simulink model "zbiornik1"  (R2015a)
settings: Solver=ode3  StartTime=0.0  StopTime=50  FixedStep=0.01  RelTol=1e-3
values from neighbouring files (symbols this model uses):
  a = 35    [ident1.m]    (also in wyniki_akt.mat; zbiornik_1.m; zbiornik_2.m; zbiornik_3.m)
  a1 = x(2)    [ident1.m]    (also in wyniki_akt.mat = 0.5)
  C1 = x(1)    [ident1.m]    (also in wyniki_akt.mat = 30)
  h10 = max(y1)    [ucinanie.m]
  w = 5    [ident1.m]    (also in wyniki_akt.mat; zbiornik_1.m; zbiornik_2.m; zbiornik_3.m)
settings Model: Creator=Ziger  LastModifiedBy=Student

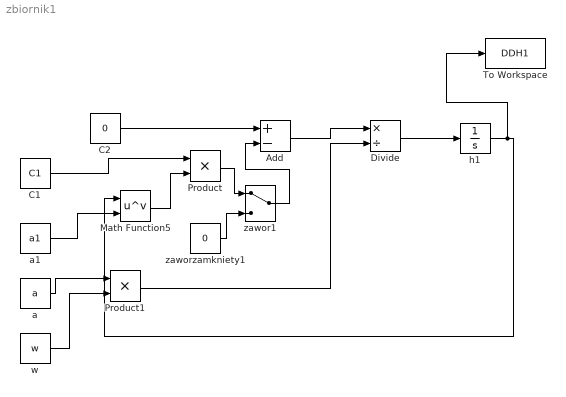
== system zbiornik1 ==
  Add : Sum  Inputs=+-
  C1 : Constant  Value=C1
  C2 : Constant  Value=0
  Divide : Product  Inputs=*/
  Math Function5 : Math  Operator=pow  SaturateOnIntegerOverflow=on
  Product : Product
  Product1 : Product
  To Workspace : ToWorkspace  VariableName=DDH1  SaveFormat=Structure With Time  SampleTime=-1
  a : Constant  Value=a
  a1 : Constant  Value=a1
  h1 : Integrator  InitialCondition=h10  LimitOutput=on  UpperSaturationLimit=35  LowerSaturationLimit=0
  w : Constant  Value=w
  "zawor1 " : ManualSwitch
  zaworzamkniety1 : Constant  Value=0
  wires:
  h1/1 -> To Workspace/1, Math Function5/1
  Add/1 -> Divide/1
  Product/1 -> "zawor1 "/1
  C1/1 -> Product/1
  a/1 -> Product1/1
  Product1/1 -> Divide/2
  w/1 -> Product1/2
  zaworzamkniety1/1 -> "zawor1 "/2
  "zawor1 "/1 -> Add/2
  Divide/1 -> h1/1
  a1/1 -> Math Function5/2
  Math Function5/1 -> Product/2
  C2/1 -> Add/1
